simulink model "system_sim_test1"  (R2015a)
settings: Solver=ode3  StartTime=0.0  StopTime=30  FixedStep=0.1  RelTol=1e-3
libraries: simulink x1
settings Model: Creator=marco  LastModifiedBy=marco

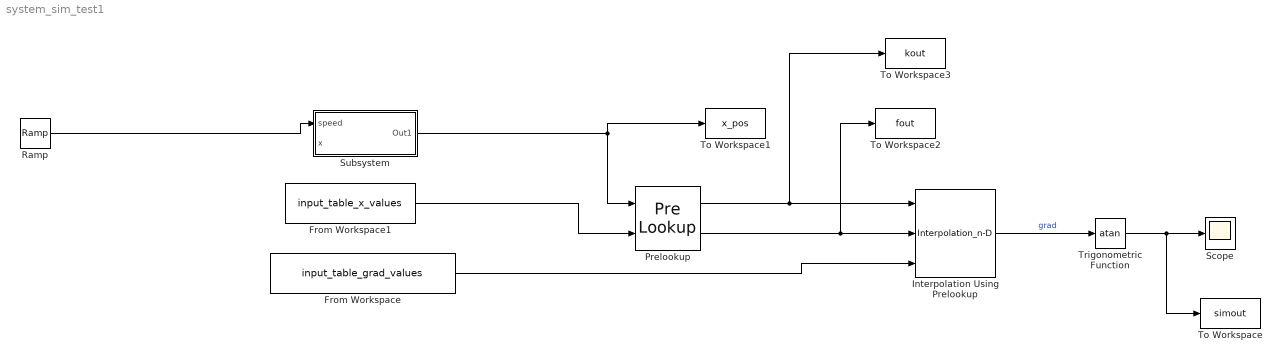
== system system_sim_test1 ==
  From Workspace : FromWorkspace  VariableName=input_table_grad_values  SampleTime=0
  From Workspace1 : FromWorkspace  VariableName=input_table_x_values  SampleTime=0
  Interpolation Using Prelookup : Interpolation_n-D  NumberOfTableDimensions=1  TableSource=Input port  InternalRulePriority=Speed
      settings: InputPortMap=u0,u1,p2
  Prelookup : PreLookup  BreakpointsDataSource=Input port  BreakpointsData=[10:10:110]  IndexSearchMethod=Linear search  ExtrapMethod=Linear
      settings: InputPortMap=u0,p1
  Ramp : simulink/Sources/Ramp  slope=1  start=0  X0=0
  Scope : Scope
  Subsystem : Subsystem
  To Workspace : ToWorkspace  VariableName=simout  SampleTime=-1
      settings: Save2DSignal=2-D array (concatenate along first dimension)
  To Workspace1 : ToWorkspace  VariableName=x_pos  SampleTime=-1
      settings: Save2DSignal=2-D array (concatenate along first dimension)
  To Workspace2 : ToWorkspace  VariableName=fout  SampleTime=-1
      settings: Save2DSignal=2-D array (concatenate along first dimension)
  To Workspace3 : ToWorkspace  VariableName=kout  SampleTime=-1
      settings: Save2DSignal=2-D array (concatenate along first dimension)
  Trigonometric Function : Trigonometry  Operator=atan
  wires:
  Interpolation Using Prelookup/1 -> Trigonometric Function/1  "grad"
  Prelookup/1 -> To Workspace3/1, Interpolation Using Prelookup/1
  Prelookup/2 -> To Workspace2/1, Interpolation Using Prelookup/2
  From Workspace/1 -> Interpolation Using Prelookup/3
  From Workspace1/1 -> Prelookup/2
  Trigonometric Function/1 -> To Workspace/1, Scope/1
  Ramp/1 -> Subsystem/1("speed ")
  Subsystem/1(Out1) -> Prelookup/1, To Workspace1/1

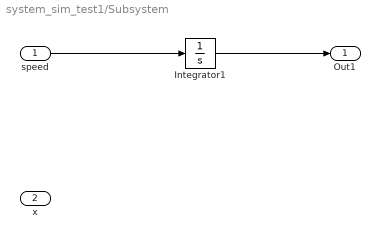
== system system_sim_test1/Subsystem ==
  "speed " : Inport
  x : Inport  Port=2
  Integrator1 : Integrator
  Out1 : Outport
  wires:
  "speed "/1 -> Integrator1/1
  Integrator1/1 -> Out1/1
